simulink library "tp333079"  (Simulink 5.0)
values from neighbouring files (symbols this model uses):
  b = 1    [main_flock3.m]    (also in main_flock4.m; params_flocking_ros.m)
undefined symbols (not defined in the file or in its folder): AC, AlphaBnd, BetaBnd, CDda, CDde, CDdf, CDdr, CDM, CDmin, CGempty, CGgross, CL0, CLa, CLalphadot, Clbeta, Clda, CLde, CLdf, Cldr, CLM, CLmind, Clp, CLq, Clr, Cm0, Cma, Cmalphadot, Cmde, Cmdf, CmM, Cmq, Cnbeta, Cnda, Cndr, Cnp, Cnr, CP, CT, CYbeta, CYda, CYdr, CYp, CYr, Displacement, dmy, Engine, EulerIni, FuelFlow, FuelIni, J, Jempty, Jeng, Jgross, Jprop, MAC, MAP, MAPLim, MassIni, MaxPower, mempty ... (+26)
libraries: aerosimlib x325, simulink3 x42
(part 10 of 11)

== system tp333079/FlightGear-Compatible/Complete Aircraft/CESSNA-182/Aerodynamics/Yaw ==
  Control : Inport  Port=1  PortDimensions=[4 1]  SampleTime=-1  DataType=auto
      settings: SignalType=auto
  WindAxesVel : Inport  Port=2  PortDimensions=[3 1]  SampleTime=-1  DataType=auto
      settings: SignalType=auto
  AngularRates : Inport  Port=3  PortDimensions=[3 1]  SampleTime=-1  DataType=auto
      settings: SignalType=auto
  2 : Gain  Gain=2  Multiplication=Element-wise(K.*u)  SaturateOnIntegerOverflow=on
  Cn aileron : Subsystem  BlockChoice=Vector  SimViewingDevice=off
      link override Value: Value=AC.Aerodynamics.Yaw.Cnda
      link override Vector: Vector=AC.Aerodynamics.Yaw.CnDa
      settings: AttributesFormatString=%<BlockChoice>  TemplateBlock=aerosimlib/FlightGear-Compatible/Aerodynamics/Coefficient  MemberBlocks=Table,Value,Vector  Permissions=ReadWrite  RTWFcnNameOpts=Auto  RTWFileNameOpts=Auto
  Cn beta : Subsystem  BlockChoice=Vector  SimViewingDevice=off
      link override Value: Value=AC.Aerodynamics.Lift.Basic.kCLge
      link override Vector: Vector=AC.Aerodynamics.Yaw.Cnb
      settings: AttributesFormatString=%<BlockChoice>  TemplateBlock=aerosimlib/FlightGear-Compatible/Aerodynamics/Coefficient  MemberBlocks=Table,Value,Vector  Permissions=ReadWrite  RTWFcnNameOpts=Auto  RTWFileNameOpts=Auto
  Cn rudder : Subsystem  BlockChoice=Vector  SimViewingDevice=off
      link override Value: Value=AC.Aerodynamics.Yaw.Cndr
      link override Vector: Vector=AC.Aerodynamics.Yaw.CnDr
      settings: AttributesFormatString=%<BlockChoice>  TemplateBlock=aerosimlib/FlightGear-Compatible/Aerodynamics/Coefficient  MemberBlocks=Table,Value,Vector  Permissions=ReadWrite  RTWFcnNameOpts=Auto  RTWFileNameOpts=Auto
  Cn*b/(2V) : Product  Inputs=**/  Multiplication=Element-wise(.*)  SaturateOnIntegerOverflow=on
  Cnb*b{,1..4} (5 alike) : Product  Inputs=2  Multiplication=Element-wise(.*)  SaturateOnIntegerOverflow=on
  Cnp : Subsystem  BlockChoice=Vector  SimViewingDevice=off
      link override Value: Value=AC.Aerodynamics.Yaw.Cnp
      link override Vector: Vector=AC.Aerodynamics.Yaw.Cnp
      settings: AttributesFormatString=%<BlockChoice>  TemplateBlock=aerosimlib/FlightGear-Compatible/Aerodynamics/Coefficient  MemberBlocks=Table,Value,Vector  Permissions=ReadWrite  RTWFcnNameOpts=Auto  RTWFileNameOpts=Auto
  Cnr : Subsystem  BlockChoice=Vector  SimViewingDevice=off
      link override Value: Value=AC.Aerodynamics.Yaw.Cnr
      link override Vector: Vector=AC.Aerodynamics.Yaw.Cnr
      settings: AttributesFormatString=%<BlockChoice>  TemplateBlock=aerosimlib/FlightGear-Compatible/Aerodynamics/Coefficient  MemberBlocks=Table,Value,Vector  Permissions=ReadWrite  RTWFcnNameOpts=Auto  RTWFileNameOpts=Auto
  Demux : Demux  Outputs=4  BusSelectionMode=off
  Demux1 : Demux  Outputs=3  BusSelectionMode=off
  Demux3 : Demux  Outputs=3  BusSelectionMode=off
  Sum : Sum  Inputs=++  SaturateOnIntegerOverflow=on
  Sum1 : Sum  Inputs=++++  SaturateOnIntegerOverflow=on
  Terminator2 : Terminator
  Terminator3 : Terminator
  Terminator4 : Terminator
  Wing span : Constant  Value=AC.Metrics.WingSpan
  Cn : Outport  Port=1
  wires:
  Demux3/3 -> Cnb*b4/2
  Demux3/1 -> Cnb*b3/2
  Demux/4 -> Cnb*b2/2
  Demux/3 -> Cnb*b1/2
  Cnb*b2/1 -> Sum1/3
  Cnb*b1/1 -> Sum1/2
  Cnb*b3/1 -> Sum/1
  Cnb*b4/1 -> Sum/2
  Cnr/1(Coeff) -> Cnb*b4/1
  Cnp/1(Coeff) -> Cnb*b3/1
  Cn rudder/1(Coeff) -> Cnb*b2/1
  Cn aileron/1(Coeff) -> Cnb*b1/1
  Demux1/2 -> Cnb*b/2
  Cn beta/1(Coeff) -> Cnb*b/1
  Cnb*b/1 -> Sum1/1
  Cn*b/(2V)/1 -> Sum1/4
  Demux/2 -> Terminator3/1
  Demux/1 -> Terminator2/1
  Demux1/3 -> Cnp/1(RowParam), Cnr/1(RowParam), Cn rudder/1(RowParam), Cn aileron/1(RowParam), Cn beta/1(RowParam)
  Demux3/2 -> Terminator4/1
  Demux1/1 -> 2/1
  Sum/1 -> Cn*b/(2V)/1
  2/1 -> Cn*b/(2V)/3
  Wing span/1 -> Cn*b/(2V)/2
  WindAxesVel/1 -> Demux1/1
  Control/1 -> Demux/1
  AngularRates/1 -> Demux3/1
  Sum1/1 -> Cn/1

== system tp333079/FlightGear-Compatible/Complete Aircraft/CESSNA-310/Aerodynamics/Drag ==
  Control : Inport  Port=1  PortDimensions=[4 1]  SampleTime=-1  DataType=auto
      settings: SignalType=auto
  WindAxesVel : Inport  Port=2  PortDimensions=[3 1]  SampleTime=-1  DataType=auto
      settings: SignalType=auto
  Gear : Inport  Port=3  PortDimensions=1  SampleTime=-1  DataType=auto
      settings: SignalType=auto
  CD alpha : Subsystem  BlockChoice=Vector  SimViewingDevice=off
      link override Table: Table=AC.Aerodynamics.Drag.Basic.CDwbh
      link override Value: Value=AC.Aerodynamics.Lift.Basic.kCLge
      link override Vector: Vector=AC.Aerodynamics.Drag.CDalpha
      settings: AttributesFormatString=%<BlockChoice>  TemplateBlock=aerosimlib/FlightGear-Compatible/Aerodynamics/Coefficient  MemberBlocks=Table,Value,Vector  Permissions=ReadWrite  RTWFcnNameOpts=Auto  RTWFileNameOpts=Auto
  CD beta : Subsystem  BlockChoice=Value  SimViewingDevice=off
      link override Value: Value=AC.Aerodynamics.Drag.CDbeta
      settings: AttributesFormatString=%<BlockChoice>  TemplateBlock=aerosimlib/FlightGear-Compatible/Aerodynamics/Coefficient  MemberBlocks=Table,Value,Vector  Permissions=ReadWrite  RTWFcnNameOpts=Auto  RTWFileNameOpts=Auto
  CD elevator : Subsystem  BlockChoice=Value  SimViewingDevice=off
      link override Value: Value=AC.Aerodynamics.Drag.CDDe
      settings: AttributesFormatString=%<BlockChoice>  TemplateBlock=aerosimlib/FlightGear-Compatible/Aerodynamics/Coefficient  MemberBlocks=Table,Value,Vector  Permissions=ReadWrite  RTWFcnNameOpts=Auto  RTWFileNameOpts=Auto
  CD flap : Subsystem  BlockChoice=Vector  SimViewingDevice=off
      link override Table: Table=AC.Aerodynamics.Drag.CDDf
      link override Value: Value=AC.Aerodynamics.Lift.Basic.kCLge
      link override Vector: Vector=AC.Aerodynamics.Drag.CDDf
      settings: AttributesFormatString=%<BlockChoice>  TemplateBlock=aerosimlib/FlightGear-Compatible/Aerodynamics/Coefficient  MemberBlocks=Table,Value,Vector  Permissions=ReadWrite  RTWFcnNameOpts=Auto  RTWFileNameOpts=Auto
  CD gear : Subsystem  BlockChoice=Value  SimViewingDevice=off
      link override Value: Value=AC.Aerodynamics.Drag.CDgear
      settings: AttributesFormatString=%<BlockChoice>  TemplateBlock=aerosimlib/FlightGear-Compatible/Aerodynamics/Coefficient  MemberBlocks=Table,Value,Vector  Permissions=ReadWrite  RTWFcnNameOpts=Auto  RTWFileNameOpts=Auto
  CDo : Constant  Value=AC.Aerodynamics.Drag.CDo.Data
  Demux : Demux  Outputs=4  BusSelectionMode=off
  Demux1 : Demux  Outputs=3  BusSelectionMode=off
  Sum : Sum  Inputs=++  SaturateOnIntegerOverflow=on
  Sum1 : Sum  Inputs=+++++  SaturateOnIntegerOverflow=on
  Terminator : Terminator
  Terminator1 : Terminator
  Terminator5 : Terminator
  CD : Outport  Port=1
  wires:
  Gear/1 -> CD gear/1(RowParam)
  CD gear/1(Coeff) -> Sum1/5
  Demux/2 -> CD elevator/1(RowParam)
  WindAxesVel/1 -> Demux1/1
  Control/1 -> Demux/1
  Demux/3 -> Terminator/1
  Demux/4 -> Terminator1/1
  Demux1/3 -> CD alpha/1(RowParam)
  CD alpha/1(Coeff) -> Sum/1
  CD flap/1(Coeff) -> Sum/2
  Sum/1 -> Sum1/1
  CDo/1 -> Sum1/2
  CD elevator/1(Coeff) -> Sum1/3
  Sum1/1 -> CD/1
  Demux1/1 -> Terminator5/1
  Demux1/2 -> CD beta/1(RowParam)
  Demux/1 -> CD flap/1(RowParam)
  CD beta/1(Coeff) -> Sum1/4

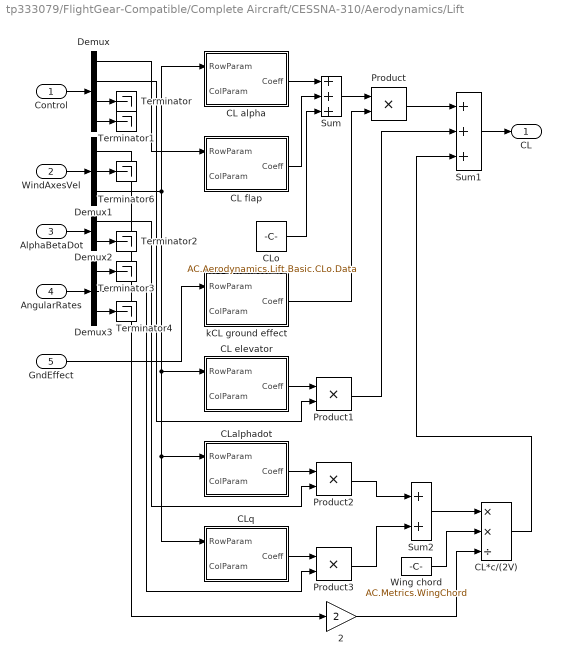
== system tp333079/FlightGear-Compatible/Complete Aircraft/CESSNA-310/Aerodynamics/Lift ==
  Control : Inport  Port=1  PortDimensions=[4 1]  SampleTime=-1  DataType=auto
      settings: SignalType=auto
  WindAxesVel : Inport  Port=2  PortDimensions=[3 1]  SampleTime=-1  DataType=auto
      settings: SignalType=auto
  AlphaBetaDot : Inport  Port=3  PortDimensions=[2 1]  SampleTime=-1  DataType=auto
      settings: SignalType=auto
  AngularRates : Inport  Port=4  PortDimensions=[3 1]  SampleTime=-1  DataType=auto
      settings: SignalType=auto
  GndEffect : Inport  Port=5  PortDimensions=1  SampleTime=-1  DataType=auto
      settings: SignalType=auto
  2 : Gain  Gain=2  Multiplication=Element-wise(K.*u)  SaturateOnIntegerOverflow=on
  CL alpha : Subsystem  BlockChoice=Vector  SimViewingDevice=off
      link override Table: Table=AC.Aerodynamics.Lift.Basic.CLalpha
      link override Value: Value=AC.Aerodynamics.Lift.Basic.kCLge
      link override Vector: Vector=AC.Aerodynamics.Lift.Basic.CLalpha
      settings: AttributesFormatString=%<BlockChoice>  TemplateBlock=aerosimlib/FlightGear-Compatible/Aerodynamics/Coefficient  MemberBlocks=Table,Value,Vector  Permissions=ReadWrite  RTWFcnNameOpts=Auto  RTWFileNameOpts=Auto
  CL elevator : Subsystem  BlockChoice=Vector  SimViewingDevice=off
      link override Value: Value=AC.Aerodynamics.Lift.CLDe
      link override Vector: Vector=AC.Aerodynamics.Lift.CLDe
      settings: AttributesFormatString=%<BlockChoice>  TemplateBlock=aerosimlib/FlightGear-Compatible/Aerodynamics/Coefficient  MemberBlocks=Table,Value,Vector  Permissions=ReadWrite  RTWFcnNameOpts=Auto  RTWFileNameOpts=Auto
  CL flap : Subsystem  BlockChoice=Vector  SimViewingDevice=off
      link override Value: Value=AC.Aerodynamics.Lift.Basic.kCLge
      link override Vector: Vector=AC.Aerodynamics.Lift.Basic.CLDf
      settings: AttributesFormatString=%<BlockChoice>  TemplateBlock=aerosimlib/FlightGear-Compatible/Aerodynamics/Coefficient  MemberBlocks=Table,Value,Vector  Permissions=ReadWrite  RTWFcnNameOpts=Auto  RTWFileNameOpts=Auto
  CL*c/(2V) : Product  Inputs=**/  Multiplication=Element-wise(.*)  SaturateOnIntegerOverflow=on
  CLalphadot : Subsystem  BlockChoice=Vector  SimViewingDevice=off
      link override Value: Value=AC.Aerodynamics.Lift.CLadot
      link override Vector: Vector=AC.Aerodynamics.Lift.CLadot
      settings: AttributesFormatString=%<BlockChoice>  TemplateBlock=aerosimlib/FlightGear-Compatible/Aerodynamics/Coefficient  MemberBlocks=Table,Value,Vector  Permissions=ReadWrite  RTWFcnNameOpts=Auto  RTWFileNameOpts=Auto
  CLo : Constant  Value=AC.Aerodynamics.Lift.Basic.CLo.Data
  CLq : Subsystem  BlockChoice=Vector  SimViewingDevice=off
      link override Value: Value=AC.Aerodynamics.Lift.CLq
      link override Vector: Vector=AC.Aerodynamics.Lift.CLq
      settings: AttributesFormatString=%<BlockChoice>  TemplateBlock=aerosimlib/FlightGear-Compatible/Aerodynamics/Coefficient  MemberBlocks=Table,Value,Vector  Permissions=ReadWrite  RTWFcnNameOpts=Auto  RTWFileNameOpts=Auto
  Demux : Demux  Outputs=4  BusSelectionMode=off
  Demux1 : Demux  Outputs=3  BusSelectionMode=off
  Demux2 : Demux  Outputs=2  BusSelectionMode=off
  Demux3 : Demux  Outputs=3  BusSelectionMode=off
  Product{,1..3} (4 alike) : Product  Inputs=2  Multiplication=Element-wise(.*)  SaturateOnIntegerOverflow=on
  Sum : Sum  Inputs=+++  SaturateOnIntegerOverflow=on
  Sum1 : Sum  Inputs=+++  SaturateOnIntegerOverflow=on
  Sum2 : Sum  Inputs=++  SaturateOnIntegerOverflow=on
  Terminator{,1..4,6} (6 alike) : Terminator
  Wing chord : Constant  Value=AC.Metrics.WingChord
  kCL ground effect : Subsystem  BlockChoice=Vector  SimViewingDevice=off
      link override Value: Value=AC.Aerodynamics.Lift.Basic.kCLge
      link override Vector: Vector=AC.Aerodynamics.Lift.Basic.kCLge
      settings: AttributesFormatString=%<BlockChoice>  TemplateBlock=aerosimlib/FlightGear-Compatible/Aerodynamics/Coefficient  MemberBlocks=Table,Value,Vector  Permissions=ReadWrite  RTWFcnNameOpts=Auto  RTWFileNameOpts=Auto
  CL : Outport  Port=1
  wires:
  Demux3/2 -> Product3/2
  Demux2/1 -> Product2/2
  Demux/2 -> Product1/2
  Product1/1 -> Sum1/2
  Product2/1 -> Sum2/1
  Product3/1 -> Sum2/2
  CLq/1(Coeff) -> Product3/1
  CLalphadot/1(Coeff) -> Product2/1
  CL elevator/1(Coeff) -> Product1/1
  CLo/1 -> Sum/3
  CL*c/(2V)/1 -> Sum1/3
  Sum2/1 -> CL*c/(2V)/1
  Wing chord/1 -> CL*c/(2V)/2
  2/1 -> CL*c/(2V)/3
  GndEffect/1 -> kCL ground effect/1(RowParam)
  Demux1/2 -> Terminator6/1
  Demux1/1 -> 2/1
  Sum1/1 -> CL/1
  Product/1 -> Sum1/1
  kCL ground effect/1(Coeff) -> Product/2
  Sum/1 -> Product/1
  CL flap/1(Coeff) -> Sum/2
  CL alpha/1(Coeff) -> Sum/1
  Demux3/3 -> Terminator4/1
  Demux3/1 -> Terminator3/1
  Demux2/2 -> Terminator2/1
  Demux1/3 -> CLq/1(RowParam), CLalphadot/1(RowParam), CL elevator/1(RowParam), CL alpha/1(RowParam)
  Demux/4 -> Terminator1/1
  Demux/3 -> Terminator/1
  Demux/1 -> CL flap/1(RowParam)
  AngularRates/1 -> Demux3/1
  AlphaBetaDot/1 -> Demux2/1
  Control/1 -> Demux/1
  WindAxesVel/1 -> Demux1/1

== system tp333079/FlightGear-Compatible/Complete Aircraft/CESSNA-310/Aerodynamics/Pitch ==
  Control : Inport  Port=1  PortDimensions=[4 1]  SampleTime=-1  DataType=auto
      settings: SignalType=auto
  WindAxesVel : Inport  Port=2  PortDimensions=[3 1]  SampleTime=-1  DataType=auto
      settings: SignalType=auto
  AlphaBetaDot : Inport  Port=3  PortDimensions=[2 1]  SampleTime=-1  DataType=auto
      settings: SignalType=auto
  AngularRates : Inport  Port=4  PortDimensions=[3 1]  SampleTime=-1  DataType=auto
      settings: SignalType=auto
  2 : Gain  Gain=2  Multiplication=Element-wise(K.*u)  SaturateOnIntegerOverflow=on
  Cm alpha : Subsystem  BlockChoice=Value  SimViewingDevice=off
      link override Table: Table=AC.Aerodynamics.Lift.Basic.CLwbh
      link override Value: Value=AC.Aerodynamics.Pitch.Cmalpha
      link override Vector: Vector=AC.Aerodynamics.Pitch.Cmalpha
      settings: AttributesFormatString=%<BlockChoice>  TemplateBlock=aerosimlib/FlightGear-Compatible/Aerodynamics/Coefficient  MemberBlocks=Table,Value,Vector  Permissions=ReadWrite  RTWFcnNameOpts=Auto  RTWFileNameOpts=Auto
  Cm elevator : Subsystem  BlockChoice=Value  SimViewingDevice=off
      link override Value: Value=AC.Aerodynamics.Pitch.CmDe
      link override Vector: Vector=AC.Aerodynamics.Pitch.CmDe
      settings: AttributesFormatString=%<BlockChoice>  TemplateBlock=aerosimlib/FlightGear-Compatible/Aerodynamics/Coefficient  MemberBlocks=Table,Value,Vector  Permissions=ReadWrite  RTWFcnNameOpts=Auto  RTWFileNameOpts=Auto
  Cm flap : Subsystem  BlockChoice=Vector  SimViewingDevice=off
      link override Value: Value=AC.Aerodynamics.Lift.Basic.kCLge
      link override Vector: Vector=AC.Aerodynamics.Pitch.CmDf
      settings: AttributesFormatString=%<BlockChoice>  TemplateBlock=aerosimlib/FlightGear-Compatible/Aerodynamics/Coefficient  MemberBlocks=Table,Value,Vector  Permissions=ReadWrite  RTWFcnNameOpts=Auto  RTWFileNameOpts=Auto
  Cm*c/(2V) : Product  Inputs=**/  Multiplication=Element-wise(.*)  SaturateOnIntegerOverflow=on
  Cmalphadot : Subsystem  BlockChoice=Value  SimViewingDevice=off
      link override Value: Value=AC.Aerodynamics.Pitch.Cmadot
      link override Vector: Vector=AC.Aerodynamics.Pitch.Cmadot
      settings: AttributesFormatString=%<BlockChoice>  TemplateBlock=aerosimlib/FlightGear-Compatible/Aerodynamics/Coefficient  MemberBlocks=Table,Value,Vector  Permissions=ReadWrite  RTWFcnNameOpts=Auto  RTWFileNameOpts=Auto
  Cmo : Constant  Value=AC.Aerodynamics.Pitch.Cmo.Data
  Cmq : Subsystem  BlockChoice=Value  SimViewingDevice=off
      link override Value: Value=AC.Aerodynamics.Pitch.Cmq
      link override Vector: Vector=AC.Aerodynamics.Pitch.Cmq
      settings: AttributesFormatString=%<BlockChoice>  TemplateBlock=aerosimlib/FlightGear-Compatible/Aerodynamics/Coefficient  MemberBlocks=Table,Value,Vector  Permissions=ReadWrite  RTWFcnNameOpts=Auto  RTWFileNameOpts=Auto
  Demux : Demux  Outputs=4  BusSelectionMode=off
  Demux1 : Demux  Outputs=3  BusSelectionMode=off
  Demux2 : Demux  Outputs=2  BusSelectionMode=off
  Demux3 : Demux  Outputs=3  BusSelectionMode=off
  Sum1 : Sum  Inputs=+++++  SaturateOnIntegerOverflow=on
  Sum2 : Sum  Inputs=++  SaturateOnIntegerOverflow=on
  Terminator{,1..4,6} (6 alike) : Terminator
  Wing chord : Constant  Value=AC.Metrics.WingChord
  Cm : Outport  Port=1
  wires:
  Cm elevator/1(Coeff) -> Sum1/4
  Cm alpha/1(Coeff) -> Sum1/1
  Cm*c/(2V)/1 -> Sum1/5
  Cmo/1 -> Sum1/3
  Cm flap/1(Coeff) -> Sum1/2
  Demux1/3 -> Cm alpha/1(RowParam)
  Demux1/1 -> 2/1
  Demux/1 -> Cm flap/1(RowParam)
  WindAxesVel/1 -> Demux1/1
  Control/1 -> Demux/1
  AlphaBetaDot/1 -> Demux2/1
  AngularRates/1 -> Demux3/1
  Demux/3 -> Terminator/1
  Demux/4 -> Terminator1/1
  Demux2/2 -> Terminator2/1
  Demux3/1 -> Terminator3/1
  Demux3/3 -> Terminator4/1
  Sum1/1 -> Cm/1
  Demux1/2 -> Terminator6/1
  2/1 -> Cm*c/(2V)/3
  Wing chord/1 -> Cm*c/(2V)/2
  Sum2/1 -> Cm*c/(2V)/1
  Demux/2 -> Cm elevator/1(RowParam)
  Cmalphadot/1(Coeff) -> Sum2/1
  Cmq/1(Coeff) -> Sum2/2
  Demux2/1 -> Cmalphadot/1(RowParam)
  Demux3/2 -> Cmq/1(RowParam)

== system tp333079/FlightGear-Compatible/Complete Aircraft/CESSNA-310/Aerodynamics/Roll ==
  Control : Inport  Port=1  PortDimensions=[4 1]  SampleTime=-1  DataType=auto
      settings: SignalType=auto
  WindAxesVel : Inport  Port=2  PortDimensions=[3 1]  SampleTime=-1  DataType=auto
      settings: SignalType=auto
  AngularRates : Inport  Port=3  PortDimensions=[3 1]  SampleTime=-1  DataType=auto
      settings: SignalType=auto
  2 : Gain  Gain=2  Multiplication=Element-wise(K.*u)  SaturateOnIntegerOverflow=on
  Cl aileron : Subsystem  BlockChoice=Value  SimViewingDevice=off
      link override Value: Value=AC.Aerodynamics.Roll.ClDa
      settings: AttributesFormatString=%<BlockChoice>  TemplateBlock=aerosimlib/FlightGear-Compatible/Aerodynamics/Coefficient  MemberBlocks=Table,Value,Vector  Permissions=ReadWrite  RTWFcnNameOpts=Auto  RTWFileNameOpts=Auto
  Cl beta : Subsystem  BlockChoice=Vector  SimViewingDevice=off
      link override Table: Table=AC.Aerodynamics.Roll.Clbeta
      link override Value: Value=AC.Aerodynamics.Lift.Basic.kCLge
      link override Vector: Vector=AC.Aerodynamics.Roll.Clbeta
      settings: AttributesFormatString=%<BlockChoice>  TemplateBlock=aerosimlib/FlightGear-Compatible/Aerodynamics/Coefficient  MemberBlocks=Table,Value,Vector  Permissions=ReadWrite  RTWFcnNameOpts=Auto  RTWFileNameOpts=Auto
  Cl rudder : Subsystem  BlockChoice=Value  SimViewingDevice=off
      link override Value: Value=AC.Aerodynamics.Roll.Cldr
      settings: AttributesFormatString=%<BlockChoice>  TemplateBlock=aerosimlib/FlightGear-Compatible/Aerodynamics/Coefficient  MemberBlocks=Table,Value,Vector  Permissions=ReadWrite  RTWFcnNameOpts=Auto  RTWFileNameOpts=Auto
  Cl*b/(2V) : Product  Inputs=**/  Multiplication=Element-wise(.*)  SaturateOnIntegerOverflow=on
  Clp : Subsystem  BlockChoice=Value  SimViewingDevice=off
      link override Value: Value=AC.Aerodynamics.Roll.Clp
      link override Vector: Vector=AC.Aerodynamics.Roll.Clp
      settings: AttributesFormatString=%<BlockChoice>  TemplateBlock=aerosimlib/FlightGear-Compatible/Aerodynamics/Coefficient  MemberBlocks=Table,Value,Vector  Permissions=ReadWrite  RTWFcnNameOpts=Auto  RTWFileNameOpts=Auto
  Clr : Subsystem  BlockChoice=Value  SimViewingDevice=off
      link override Value: Value=AC.Aerodynamics.Roll.Clr
      link override Vector: Vector=AC.Aerodynamics.Roll.Clr
      settings: AttributesFormatString=%<BlockChoice>  TemplateBlock=aerosimlib/FlightGear-Compatible/Aerodynamics/Coefficient  MemberBlocks=Table,Value,Vector  Permissions=ReadWrite  RTWFcnNameOpts=Auto  RTWFileNameOpts=Auto
  Demux : Demux  Outputs=4  BusSelectionMode=off
  Demux1 : Demux  Outputs=3  BusSelectionMode=off
  Demux3 : Demux  Outputs=3  BusSelectionMode=off
  Sum : Sum  Inputs=++  SaturateOnIntegerOverflow=on
  Sum1 : Sum  Inputs=++++  SaturateOnIntegerOverflow=on
  Terminator2 : Terminator
  Terminator3 : Terminator
  Terminator4 : Terminator
  Wing span : Constant  Value=AC.Metrics.WingSpan
  Cl : Outport  Port=1
  wires:
  Clr/1(Coeff) -> Sum/2
  Clp/1(Coeff) -> Sum/1
  Sum1/1 -> Cl/1
  AngularRates/1 -> Demux3/1
  Control/1 -> Demux/1
  WindAxesVel/1 -> Demux1/1
  Wing span/1 -> Cl*b/(2V)/2
  2/1 -> Cl*b/(2V)/3
  Sum/1 -> Cl*b/(2V)/1
  Demux1/1 -> 2/1
  Demux1/2 -> Cl beta/1(RowParam)
  Demux/3 -> Cl aileron/1(RowParam)
  Demux/4 -> Cl rudder/1(RowParam)
  Demux3/2 -> Terminator4/1
  Demux/1 -> Terminator2/1
  Demux/2 -> Terminator3/1
  Cl beta/1(Coeff) -> Sum1/1
  Cl aileron/1(Coeff) -> Sum1/2
  Cl rudder/1(Coeff) -> Sum1/3
  Cl*b/(2V)/1 -> Sum1/4
  Demux3/1 -> Clp/1(RowParam)
  Demux3/3 -> Clr/1(RowParam)

== system tp333079/FlightGear-Compatible/Complete Aircraft/CESSNA-310/Aerodynamics/Side ==
  Control : Inport  Port=1  PortDimensions=[4 1]  SampleTime=-1  DataType=auto
      settings: SignalType=auto
  WindAxesVel : Inport  Port=2  PortDimensions=[3 1]  SampleTime=-1  DataType=auto
      settings: SignalType=auto
  AngularRates : Inport  Port=3  PortDimensions=[3 1]  SampleTime=-1  DataType=auto
      settings: SignalType=auto
  2 : Gain  Gain=2  Multiplication=Element-wise(K.*u)  SaturateOnIntegerOverflow=on
  CY beta : Subsystem  BlockChoice=Vector  SimViewingDevice=off
      link override Value: Value=AC.Aerodynamics.Lift.Basic.kCLge
      link override Vector: Vector=AC.Aerodynamics.Side.CYbeta
      settings: AttributesFormatString=%<BlockChoice>  TemplateBlock=aerosimlib/FlightGear-Compatible/Aerodynamics/Coefficient  MemberBlocks=Table,Value,Vector  Permissions=ReadWrite  RTWFcnNameOpts=Auto  RTWFileNameOpts=Auto
  CY rudder : Subsystem  BlockChoice=Value  SimViewingDevice=off
      link override Value: Value=AC.Aerodynamics.Side.CYDr
      settings: AttributesFormatString=%<BlockChoice>  TemplateBlock=aerosimlib/FlightGear-Compatible/Aerodynamics/Coefficient  MemberBlocks=Table,Value,Vector  Permissions=ReadWrite  RTWFcnNameOpts=Auto  RTWFileNameOpts=Auto
  CY*b/(2V) : Product  Inputs=**/  Multiplication=Element-wise(.*)  SaturateOnIntegerOverflow=on
  CYp : Subsystem  BlockChoice=Value  SimViewingDevice=off
      link override Value: Value=AC.Aerodynamics.Side.CYp
      link override Vector: Vector=AC.Aerodynamics.Side.CYp
      settings: AttributesFormatString=%<BlockChoice>  TemplateBlock=aerosimlib/FlightGear-Compatible/Aerodynamics/Coefficient  MemberBlocks=Table,Value,Vector  Permissions=ReadWrite  RTWFcnNameOpts=Auto  RTWFileNameOpts=Auto
  CYr : Subsystem  BlockChoice=Value  SimViewingDevice=off
      link override Value: Value=AC.Aerodynamics.Side.CYr
      link override Vector: Vector=AC.Aerodynamics.Side.CYr
      settings: AttributesFormatString=%<BlockChoice>  TemplateBlock=aerosimlib/FlightGear-Compatible/Aerodynamics/Coefficient  MemberBlocks=Table,Value,Vector  Permissions=ReadWrite  RTWFcnNameOpts=Auto  RTWFileNameOpts=Auto
  Demux : Demux  Outputs=4  BusSelectionMode=off
  Demux1 : Demux  Outputs=3  BusSelectionMode=off
  Demux3 : Demux  Outputs=3  BusSelectionMode=off
  Sum : Sum  Inputs=++  SaturateOnIntegerOverflow=on
  Sum1 : Sum  Inputs=++++  SaturateOnIntegerOverflow=on
  Terminator2 : Terminator
  Terminator3 : Terminator
  Terminator4 : Terminator
  Wing span : Constant  Value=AC.Metrics.WingSpan
  CY : Outport  Port=1
  wires:
  Demux3/3 -> CYr/1(RowParam)
  CYr/1(Coeff) -> Sum/2
  CYp/1(Coeff) -> Sum/1
  CY*b/(2V)/1 -> Sum1/4
  CY rudder/1(Coeff) -> Sum1/3
  Demux/2 -> Terminator3/1
  Demux/1 -> Terminator2/1
  Demux3/2 -> Terminator4/1
  Demux/4 -> CY rudder/1(RowParam)
  Demux1/1 -> 2/1
  Sum/1 -> CY*b/(2V)/1
  2/1 -> CY*b/(2V)/3
  Wing span/1 -> CY*b/(2V)/2
  WindAxesVel/1 -> Demux1/1
  Control/1 -> Demux/1
  AngularRates/1 -> Demux3/1
  Sum1/1 -> CY/1
  CY beta/1(Coeff) -> Sum1/1
  Demux1/2 -> CY beta/1(RowParam)
  Demux3/1 -> CYp/1(RowParam)

== system tp333079/FlightGear-Compatible/Complete Aircraft/CESSNA-310/Aerodynamics/Yaw ==
  Control : Inport  Port=1  PortDimensions=[4 1]  SampleTime=-1  DataType=auto
      settings: SignalType=auto
  WindAxesVel : Inport  Port=2  PortDimensions=[3 1]  SampleTime=-1  DataType=auto
      settings: SignalType=auto
  AngularRates : Inport  Port=3  PortDimensions=[3 1]  SampleTime=-1  DataType=auto
      settings: SignalType=auto
  2 : Gain  Gain=2  Multiplication=Element-wise(K.*u)  SaturateOnIntegerOverflow=on
  Cn aileron : Subsystem  BlockChoice=Value  SimViewingDevice=off
      link override Value: Value=AC.Aerodynamics.Yaw.CnDa
      link override Vector: Vector=AC.Aerodynamics.Yaw.CnDa
      settings: AttributesFormatString=%<BlockChoice>  TemplateBlock=aerosimlib/FlightGear-Compatible/Aerodynamics/Coefficient  MemberBlocks=Table,Value,Vector  Permissions=ReadWrite  RTWFcnNameOpts=Auto  RTWFileNameOpts=Auto
  Cn beta : Subsystem  BlockChoice=Value  SimViewingDevice=off
      link override Value: Value=AC.Aerodynamics.Yaw.Cnbeta
      link override Vector: Vector=AC.Aerodynamics.Yaw.Cnb
      settings: AttributesFormatString=%<BlockChoice>  TemplateBlock=aerosimlib/FlightGear-Compatible/Aerodynamics/Coefficient  MemberBlocks=Table,Value,Vector  Permissions=ReadWrite  RTWFcnNameOpts=Auto  RTWFileNameOpts=Auto
  Cn rudder : Subsystem  BlockChoice=Value  SimViewingDevice=off
      link override Value: Value=AC.Aerodynamics.Yaw.CnDr
      link override Vector: Vector=AC.Aerodynamics.Yaw.CnDr
      settings: AttributesFormatString=%<BlockChoice>  TemplateBlock=aerosimlib/FlightGear-Compatible/Aerodynamics/Coefficient  MemberBlocks=Table,Value,Vector  Permissions=ReadWrite  RTWFcnNameOpts=Auto  RTWFileNameOpts=Auto
  Cn*b/(2V) : Product  Inputs=**/  Multiplication=Element-wise(.*)  SaturateOnIntegerOverflow=on
  Cnp : Subsystem  BlockChoice=Value  SimViewingDevice=off
      link override Value: Value=AC.Aerodynamics.Yaw.Cnp
      link override Vector: Vector=AC.Aerodynamics.Yaw.Cnp
      settings: AttributesFormatString=%<BlockChoice>  TemplateBlock=aerosimlib/FlightGear-Compatible/Aerodynamics/Coefficient  MemberBlocks=Table,Value,Vector  Permissions=ReadWrite  RTWFcnNameOpts=Auto  RTWFileNameOpts=Auto
  Cnr : Subsystem  BlockChoice=Value  SimViewingDevice=off
      link override Value: Value=AC.Aerodynamics.Yaw.Cnr
      link override Vector: Vector=AC.Aerodynamics.Yaw.Cnr
      settings: AttributesFormatString=%<BlockChoice>  TemplateBlock=aerosimlib/FlightGear-Compatible/Aerodynamics/Coefficient  MemberBlocks=Table,Value,Vector  Permissions=ReadWrite  RTWFcnNameOpts=Auto  RTWFileNameOpts=Auto
  Demux : Demux  Outputs=4  BusSelectionMode=off
  Demux1 : Demux  Outputs=3  BusSelectionMode=off
  Demux3 : Demux  Outputs=3  BusSelectionMode=off
  Sum : Sum  Inputs=++  SaturateOnIntegerOverflow=on
  Sum1 : Sum  Inputs=++++  SaturateOnIntegerOverflow=on
  Terminator2 : Terminator
  Terminator3 : Terminator
  Terminator4 : Terminator
  Wing span : Constant  Value=AC.Metrics.WingSpan
  Cn : Outport  Port=1
  wires:
  Demux/4 -> Cn rudder/1(RowParam)
  Cn aileron/1(Coeff) -> Sum1/2
  Cnr/1(Coeff) -> Sum/2
  Cnp/1(Coeff) -> Sum/1
  Cn rudder/1(Coeff) -> Sum1/3
  Cn*b/(2V)/1 -> Sum1/4
  Demux/2 -> Terminator3/1
  Demux/1 -> Terminator2/1
  Demux3/2 -> Terminator4/1
  Demux1/1 -> 2/1
  Sum/1 -> Cn*b/(2V)/1
  2/1 -> Cn*b/(2V)/3
  Wing span/1 -> Cn*b/(2V)/2
  WindAxesVel/1 -> Demux1/1
  Control/1 -> Demux/1
  AngularRates/1 -> Demux3/1
  Sum1/1 -> Cn/1
  Demux/3 -> Cn aileron/1(RowParam)
  Cn beta/1(Coeff) -> Sum1/1
  Demux1/2 -> Cn beta/1(RowParam)
  Demux3/1 -> Cnp/1(RowParam)
  Demux3/3 -> Cnr/1(RowParam)

== system tp333079/FlightGear-Compatible/Propulsion/Engine/Piston/AirFlow Model ==
  MAP : Inport  Port=1  PortDimensions=-1  SampleTime=-1  DataType=auto
      settings: SignalType=auto
  RPM : Inport  Port=2  PortDimensions=-1  SampleTime=-1  DataType=auto
      settings: SignalType=auto
  rho : Inport  Port=3  PortDimensions=-1  SampleTime=-1  DataType=auto
      settings: SignalType=auto
  p : Inport  Port=4  PortDimensions=-1  SampleTime=-1  DataType=auto
      settings: SignalType=auto
  1/2 : Gain  Gain=1/2  Multiplication=Element-wise(K.*u)  SaturateOnIntegerOverflow=on
  Displacement : Constant  Value=Disp/(100)^3
  Product : Product  Inputs=2  Multiplication=Element-wise(.*)  SaturateOnIntegerOverflow=on
  Product1 : Product  Inputs=3  Multiplication=Element-wise(.*)  SaturateOnIntegerOverflow=on
  Product2 : Product  Inputs=**/  Multiplication=Element-wise(.*)  SaturateOnIntegerOverflow=on
  Volumetric eff : Constant  Value=VolEff
  rot/sec : Gain  Gain=1/60  Multiplication=Element-wise(K.*u)  SaturateOnIntegerOverflow=on
  AirFlow : Outport  Port=1
  wires:
  Product1/1 -> AirFlow/1
  Product2/1 -> Product1/3
  p/1 -> Product2/3
  MAP/1 -> Product2/2
  rho/1 -> Product2/1
  Volumetric eff/1 -> Product1/2
  1/2/1 -> Product1/1
  Product/1 -> 1/2/1
  Displacement/1 -> Product/2
  rot/sec/1 -> Product/1
  RPM/1 -> rot/sec/1

== system tp333079/FlightGear-Compatible/Propulsion/Engine/Piston/FG Piston Engine ==
  Thr : Inport  Port=1  PortDimensions=1  SampleTime=-1  DataType=double
      settings: SignalType=auto
  Mix : Inport  Port=2  PortDimensions=1  SampleTime=-1  DataType=double
      settings: SignalType=auto
  Omega : Inport  Port=3  PortDimensions=1  SampleTime=-1  DataType=double
      settings: SignalType=auto
  p : Inport  Port=4  PortDimensions=1  SampleTime=-1  DataType=double
      settings: SignalType=auto
  T : Inport  Port=5  PortDimensions=1  SampleTime=-1  DataType=double
      settings: SignalType=auto
  rho : Inport  Port=6  PortDimensions=1  SampleTime=-1  DataType=double
      settings: SignalType=auto
  AirFlow Model : aerosimlib/FlightGear-Compatible/Propulsion/Engine/Piston/AirFlow Model  VolEff=0.8  Disp=Eng.Param.Displacement
  Engine torque : Product  Inputs=*/  Multiplication=Element-wise(.*)  SaturateOnIntegerOverflow=on
  Engine  BSFC : Product  Inputs=*/  Multiplication=Element-wise(.*)  SaturateOnIntegerOverflow=on
  FuelFlow Model : aerosimlib/FlightGear-Compatible/Propulsion/Engine/Piston/FuelFlow Model  pSL=pSL
  Intake Model : aerosimlib/FlightGear-Compatible/Propulsion/Engine/Piston/Intake Model  MAPLim=Eng.Param.MAPLim  pSL=pSL
  Power Model : aerosimlib/FlightGear-Compatible/Propulsion/Engine/Piston/Power Model  TSL=TSL  MaxPower=Eng.Param.MaxPower  Mixture=[14.7/1.6 10 11 12 13 14 15 16 17 18 19 20 14.7/0.6]  PowerMixCor=[78 86 93 98 100 99 96.4 92.5 88 83 78.5 74 58]
  rad/s 2 RPM : aerosimlib/Unit Conversion/Angular velocity/rad//s 2 RPM
  MAP : Outport  Port=1
  AirFlow : Outport  Port=2
  FuelFlow : Outport  Port=3
  BSFC : Outport  Port=4
  Power : Outport  Port=5
  Torque : Outport  Port=6
  wires:
  Power Model/1 -> Engine torque/1, Engine  BSFC/2, Power/1
  FuelFlow Model/2 -> FuelFlow/1, Engine  BSFC/1
  Mix/1 -> FuelFlow Model/1
  rho/1 -> AirFlow Model/3
  T/1 -> Power Model/3
  FuelFlow Model/1 -> Power Model/4
  AirFlow Model/1 -> AirFlow/1, FuelFlow Model/3
  rad/s 2 RPM/1 -> Power Model/2, AirFlow Model/2
  Intake Model/1 -> MAP/1, Power Model/1, AirFlow Model/1
  Omega/1 -> Engine torque/2, rad/s 2 RPM/1
  Engine  BSFC/1 -> BSFC/1
  Engine torque/1 -> Torque/1
  Thr/1 -> Intake Model/1
  p/1 -> AirFlow Model/4, FuelFlow Model/2, Intake Model/2

== system tp333079/FlightGear-Compatible/Propulsion/Engine/Piston/FuelFlow Model ==
  Mix : Inport  Port=1  PortDimensions=-1  SampleTime=-1  DataType=auto
      settings: SignalType=auto
  p : Inport  Port=2  PortDimensions=-1  SampleTime=-1  DataType=auto
      settings: SignalType=auto
  AirFlow : Inport  Port=3  PortDimensions=-1  SampleTime=-1  DataType=auto
      settings: SignalType=auto
  Gain : Gain  Gain=1.3  Multiplication=Element-wise(K.*u)  SaturateOnIntegerOverflow=on
  Product : Product  Inputs=**/  Multiplication=Element-wise(.*)  SaturateOnIntegerOverflow=on
  Product1 : Product  Inputs=**/  Multiplication=Element-wise(.*)  SaturateOnIntegerOverflow=on
  Sea-level pressure : Constant  Value=pSL
  coef : Constant  Value=14.7
  EquivRatio : Outport  Port=1
  FuelFlow : Outport  Port=2
  wires:
  Product1/1 -> FuelFlow/1
  coef/1 -> Product1/3
  AirFlow/1 -> Product1/2
  Product/1 -> Product1/1, EquivRatio/1
  p/1 -> Product/3
  Sea-level pressure/1 -> Product/2
  Gain/1 -> Product/1
  Mix/1 -> Gain/1

== system tp333079/FlightGear-Compatible/Propulsion/Engine/Piston/Intake Model ==
  Thr : Inport  Port=1  PortDimensions=1  SampleTime=-1  DataType=double
      settings: SignalType=auto
  p : Inport  Port=2  PortDimensions=1  SampleTime=-1  DataType=double
      settings: SignalType=auto
  Get MAP Altitude : Product  Inputs=**/  Multiplication=Element-wise(.*)  SaturateOnIntegerOverflow=on
  Get MAP Sea-level : Product  Inputs=2  Multiplication=Element-wise(.*)  SaturateOnIntegerOverflow=on
  MAP max : Constant  Value=MAPLim(2)
  MAP min : Constant  Value=MAPLim(1)
  Saturation : Saturate  UpperLimit=MAPLim(2)  LowerLimit=MAPLim(1)  LinearizeAsGain=on
  Sum : Sum  Inputs=|+-  SaturateOnIntegerOverflow=on
  Sum1 : Sum  Inputs=|++  SaturateOnIntegerOverflow=on
  p ambient : Constant  Value=pSL
  MAP : Outport  Port=1
  wires:
  Get MAP Altitude/1 -> MAP/1
  p ambient/1 -> Get MAP Altitude/3
  p/1 -> Get MAP Altitude/2
  Saturation/1 -> Get MAP Altitude/1
  MAP max/1 -> Sum/1
  Thr/1 -> Get MAP Sea-level/1
  MAP min/1 -> Sum/2, Sum1/2
  Sum/1 -> Get MAP Sea-level/2
  Get MAP Sea-level/1 -> Sum1/1
  Sum1/1 -> Saturation/1

== system tp333079/FlightGear-Compatible/Propulsion/Engine/Piston/Power Model ==
  MAP : Inport  Port=1  PortDimensions=-1  SampleTime=-1  DataType=auto
      settings: SignalType=auto
  RPM : Inport  Port=2  PortDimensions=-1  SampleTime=-1  DataType=auto
      settings: SignalType=auto
  T : Inport  Port=3  PortDimensions=-1  SampleTime=-1  DataType=auto
      settings: SignalType=auto
  EquivRatio : Inport  Port=4  PortDimensions=-1  SampleTime=-1  DataType=auto
      settings: SignalType=auto
  Gain : Gain  Gain=1/100  Multiplication=Element-wise(K.*u)  SaturateOnIntegerOverflow=on
  Gain1 : Gain  Gain=1/100  Multiplication=Element-wise(K.*u)  SaturateOnIntegerOverflow=on
  K2F : aerosimlib/Unit Conversion/Temperature/K2F
  K2F1 : aerosimlib/Unit Conversion/Temperature/K2F
  Look-Up Table : Lookup  InputValues=Mixture  OutputValues=PowerMixCor
  Math Function : Math  Operator=square  OutputSignalType=auto
  MaxPower : Constant  Value=MaxPower
  Pa2inHg : aerosimlib/Unit Conversion/Pressure/Pa2inHg
  Product{,1..3} (4 alike) : Product  Inputs=2  Multiplication=Element-wise(.*)  SaturateOnIntegerOverflow=on
  Product4 : Product  Inputs=3  Multiplication=Element-wise(.*)  SaturateOnIntegerOverflow=on
  Product5 : Product  Inputs=*/  Multiplication=Element-wise(.*)  SaturateOnIntegerOverflow=on
  Sum : Sum  Inputs=++-+  SaturateOnIntegerOverflow=on
  Sum1 : Sum  Inputs=|+-  SaturateOnIntegerOverflow=on
  T ambient : Constant  Value=TSL
  coef1 : Constant  Value=6e-9
  coef2 : Constant  Value=8e-4
  coef3 : Constant  Value=1
  coef4 : Constant  Value=7/120
  coef5 : Constant  Value=14.7
  Power : Outport  Port=1
  wires:
  coef5/1 -> Product5/1
  EquivRatio/1 -> Product5/2
  Product5/1 -> Look-Up Table/1
  Product4/1 -> Power/1
  MaxPower/1 -> Product4/3
  Gain/1 -> Product4/2
  Gain1/1 -> Product4/1
  Sum/1 -> Gain1/1
  Look-Up Table/1 -> Gain/1
  Product3/1 -> Sum/4
  coef4/1 -> Product3/2
  Sum1/1 -> Product3/1
  RPM/1 -> Product/2
  Pa2inHg/1 -> Product/1
  K2F/1 -> Sum1/2
  K2F1/1 -> Sum1/1
  T ambient/1 -> K2F1/1
  T/1 -> K2F/1
  coef3/1 -> Sum/3
  Product2/1 -> Sum/2
  Product1/1 -> Sum/1
  coef2/1 -> Product2/2
  coef1/1 -> Product1/2
  Math Function/1 -> Product1/1
  Product/1 -> Product2/1, Math Function/1
  MAP/1 -> Pa2inHg/1

== system tp333079/FlightGear-Compatible/Propulsion/Thruster/Propeller/FG Fixed-Pitch Propeller ==
  note: Sources
  note: Compute advance ratio
  note: Compute thrust force
  note: Interpolate propeller coefficients
  note: Compute torque
  Airspeed : Inport  Port=1  PortDimensions=1  SampleTime=-1  DataType=double
      settings: SignalType=auto
  rho : Inport  Port=2  PortDimensions=1  SampleTime=-1  DataType=double
      settings: SignalType=auto
  Omega : Inport  Port=3  PortDimensions=1  SampleTime=-1  DataType=double
      settings: SignalType=auto
  1/pi^2 : Math  Operator=pow  OutputSignalType=auto
  1/pi^3 : Math  Operator=pow  OutputSignalType=auto
  Advance Ratio : Product  Inputs=**//  Multiplication=Element-wise(.*)  SaturateOnIntegerOverflow=on
  Coeff of Power : Lookup  InputValues=Thr.Param.CoefPower(:,1)  OutputValues=Thr.Param.CoefPower(:,2)
  Coeff of Thrust : Lookup  InputValues=Thr.Param.CoefThrust(:,1)  OutputValues=Thr.Param.CoefThrust(:,2)
  Gain : Gain  Gain=4  Multiplication=Element-wise(K.*u)  SaturateOnIntegerOverflow=on
  Gain1 : Gain  Gain=-4  Multiplication=Element-wise(K.*u)  SaturateOnIntegerOverflow=on
  Mux : Mux  Inputs=3
  Omega^2 : Math  Operator=square  OutputSignalType=auto
  Pi : Constant  Value=pi
  Prop Radius : Constant  Value=Thr.Param.Diameter/2
  R^4 : Math  Operator=pow  OutputSignalType=auto
  R^5 : Math  Operator=pow  OutputSignalType=auto
  Thrust : Product  Inputs=5  Multiplication=Element-wise(.*)  SaturateOnIntegerOverflow=on
  Torque : Product  Inputs=5  Multiplication=Element-wise(.*)  SaturateOnIntegerOverflow=on
  exp : Constant  Value=-3
  exp1 : Constant  Value=4
  exp2 : Constant  Value=5
  exp3 : Constant  Value=-2
  Fprop : Outport  Port=1
  Mprop : Outport  Port=2
  PropCoeff : Outport  Port=3
  wires:
  exp3/1 -> 1/pi^2/2
  Coeff of Power/1 -> Mux/3, Torque/5
  Airspeed/1 -> Advance Ratio/2
  rho/1 -> Torque/2, Thrust/2
  Omega/1 -> Advance Ratio/3, Omega^2/1
  Pi/1 -> Advance Ratio/1, 1/pi^2/1, 1/pi^3/1
  Prop Radius/1 -> Advance Ratio/4, R^4/1, R^5/1
  Advance Ratio/1 -> Mux/1, Coeff of Power/1, Coeff of Thrust/1
  Omega^2/1 -> Torque/4, Thrust/4
  exp/1 -> 1/pi^3/2
  1/pi^2/1 -> Gain/1
  1/pi^3/1 -> Gain1/1
  exp1/1 -> R^4/2
  R^4/1 -> Thrust/3
  exp2/1 -> R^5/2
  R^5/1 -> Torque/3
  Gain/1 -> Thrust/1
  Gain1/1 -> Torque/1
  Coeff of Thrust/1 -> Mux/2, Thrust/5
  Thrust/1 -> Fprop/1
  Torque/1 -> Mprop/1
  Mux/1 -> PropCoeff/1

== system tp333079/FlightGear-Compatible/Propulsion/Thruster/Propeller/FG Variable-Pitch Propeller ==
  note: Sources
  note: Compute advance ratio
  note: Compute thrust force
  note: Interpolate propeller coefficients
  note: Compute torque
  Airspeed : Inport  Port=1  PortDimensions=1  SampleTime=-1  DataType=double
      settings: SignalType=auto
  rho : Inport  Port=2  PortDimensions=1  SampleTime=-1  DataType=double
      settings: SignalType=auto
  Omega : Inport  Port=3  PortDimensions=1  SampleTime=-1  DataType=double
      settings: SignalType=auto
  Pitch : Inport  Port=4  PortDimensions=1  SampleTime=-1  DataType=double
      settings: SignalType=auto
  1/pi^2 : Math  Operator=pow  OutputSignalType=auto
  1/pi^3 : Math  Operator=pow  OutputSignalType=auto
  Advance Ratio : Product  Inputs=**//  Multiplication=Element-wise(.*)  SaturateOnIntegerOverflow=on
  Coeff of Power : Lookup2D  RowIndex=Thr.Param.CoefPower(2:end,1)  ColumnIndex=Thr.Param.CoefPower(1,2:end)  OutputValues=Thr.Param.CoefPower(2:end,2:end)
  Coeff of Thrust : Lookup2D  RowIndex=Thr.Param.CoefThrust(2:end,1)  ColumnIndex=Thr.Param.CoefThrust(1,2:end)  OutputValues=Thr.Param.CoefThrust(2:end,2:end)
  Gain : Gain  Gain=4  Multiplication=Element-wise(K.*u)  SaturateOnIntegerOverflow=on
  Gain1 : Gain  Gain=-4  Multiplication=Element-wise(K.*u)  SaturateOnIntegerOverflow=on
  Mux : Mux  Inputs=3
  Omega^2 : Math  Operator=square  OutputSignalType=auto
  Pi : Constant  Value=pi
  Prop Radius : Constant  Value=Thr.Param.Diameter/2
  R^4 : Math  Operator=pow  OutputSignalType=auto
  R^5 : Math  Operator=pow  OutputSignalType=auto
  Thrust : Product  Inputs=5  Multiplication=Element-wise(.*)  SaturateOnIntegerOverflow=on
  Torque : Product  Inputs=5  Multiplication=Element-wise(.*)  SaturateOnIntegerOverflow=on
  exp : Constant  Value=-3
  exp1 : Constant  Value=4
  exp2 : Constant  Value=5
  exp3 : Constant  Value=-2
  Fprop : Outport  Port=1
  Mprop : Outport  Port=2
  PropCoeff : Outport  Port=3
  wires:
  Pitch/1 -> Coeff of Power/2, Coeff of Thrust/2
  exp3/1 -> 1/pi^2/2
  Coeff of Power/1 -> Mux/3, Torque/5
  Airspeed/1 -> Advance Ratio/2
  rho/1 -> Torque/2, Thrust/2
  Omega/1 -> Advance Ratio/3, Omega^2/1
  Pi/1 -> Advance Ratio/1, 1/pi^2/1, 1/pi^3/1
  Prop Radius/1 -> Advance Ratio/4, R^4/1, R^5/1
  Advance Ratio/1 -> Coeff of Power/1, Mux/1, Coeff of Thrust/1
  Omega^2/1 -> Torque/4, Thrust/4
  exp/1 -> 1/pi^3/2
  1/pi^2/1 -> Gain/1
  1/pi^3/1 -> Gain1/1
  exp1/1 -> R^4/2
  R^4/1 -> Thrust/3
  exp2/1 -> R^5/2
  R^5/1 -> Torque/3
  Gain/1 -> Thrust/1
  Gain1/1 -> Torque/1
  Coeff of Thrust/1 -> Mux/2, Thrust/5
  Thrust/1 -> Fprop/1
  Torque/1 -> Mprop/1
  Mux/1 -> PropCoeff/1

== system tp333079/FlightGear-Compatible/Complete Aircraft/CESSNA-172/Aerodynamics/Drag/CD alpha ==
  RowParam : Inport  Port=1  PortDimensions=-1  SampleTime=-1  DataType=auto
      settings: SignalType=auto
  ColParam : Inport  Port=2  PortDimensions=-1  SampleTime=-1  DataType=auto
      settings: SignalType=auto
  Table : aerosimlib/FlightGear-Compatible/Aerodynamics/Table  Table=AC.Aerodynamics.Drag.Basic.CDwbh
  Coeff : Outport  Port=1
  wires:
  Table/1 -> Coeff/1
  ColParam/1 -> Table/2
  RowParam/1 -> Table/1

== system tp333079/FlightGear-Compatible/Complete Aircraft/CESSNA-172/Aerodynamics/Drag/CD beta ==
  RowParam : Inport  Port=1  PortDimensions=-1  SampleTime=-1  DataType=auto
      settings: SignalType=auto
  ColParam : Inport  Port=2  PortDimensions=-1  SampleTime=-1  DataType=auto
      settings: SignalType=auto
  Value : aerosimlib/FlightGear-Compatible/Aerodynamics/Value  Value=AC.Aerodynamics.Drag.CDbeta
  term2 : Terminator
  Coeff : Outport  Port=1
  wires:
  ColParam/1 -> term2/1
  Value/1 -> Coeff/1
  RowParam/1 -> Value/1

== system tp333079/FlightGear-Compatible/Complete Aircraft/CESSNA-172/Aerodynamics/Drag/CD elevator ==
  RowParam : Inport  Port=1  PortDimensions=-1  SampleTime=-1  DataType=auto
      settings: SignalType=auto
  ColParam : Inport  Port=2  PortDimensions=-1  SampleTime=-1  DataType=auto
      settings: SignalType=auto
  Value : aerosimlib/FlightGear-Compatible/Aerodynamics/Value  Value=AC.Aerodynamics.Drag.CDDe
  term2 : Terminator
  Coeff : Outport  Port=1
  wires:
  ColParam/1 -> term2/1
  Value/1 -> Coeff/1
  RowParam/1 -> Value/1

== system tp333079/FlightGear-Compatible/Complete Aircraft/CESSNA-172/Aerodynamics/Drag/CD flap ==
  RowParam : Inport  Port=1  PortDimensions=-1  SampleTime=-1  DataType=auto
      settings: SignalType=auto
  ColParam : Inport  Port=2  PortDimensions=-1  SampleTime=-1  DataType=auto
      settings: SignalType=auto
  Vector : aerosimlib/FlightGear-Compatible/Aerodynamics/Vector  Vector=AC.Aerodynamics.Drag.Basic.CDDf
  term2 : Terminator
  Coeff : Outport  Port=1
  wires:
  ColParam/1 -> term2/1
  Vector/1 -> Coeff/1
  RowParam/1 -> Vector/1

== system tp333079/FlightGear-Compatible/Complete Aircraft/CESSNA-172/Aerodynamics/Drag/kCD ground effect ==
  RowParam : Inport  Port=1  PortDimensions=-1  SampleTime=-1  DataType=auto
      settings: SignalType=auto
  ColParam : Inport  Port=2  PortDimensions=-1  SampleTime=-1  DataType=auto
      settings: SignalType=auto
  Vector : aerosimlib/FlightGear-Compatible/Aerodynamics/Vector  Vector=AC.Aerodynamics.Drag.Basic.kCDge
  term2 : Terminator
  Coeff : Outport  Port=1
  wires:
  ColParam/1 -> term2/1
  Vector/1 -> Coeff/1
  RowParam/1 -> Vector/1

== system tp333079/FlightGear-Compatible/Complete Aircraft/CESSNA-172/Aerodynamics/Lift/CL alpha ==
  RowParam : Inport  Port=1  PortDimensions=-1  SampleTime=-1  DataType=auto
      settings: SignalType=auto
  ColParam : Inport  Port=2  PortDimensions=-1  SampleTime=-1  DataType=auto
      settings: SignalType=auto
  Table : aerosimlib/FlightGear-Compatible/Aerodynamics/Table  Table=AC.Aerodynamics.Lift.Basic.CLwbh
  Coeff : Outport  Port=1
  wires:
  RowParam/1 -> Table/1
  ColParam/1 -> Table/2
  Table/1 -> Coeff/1

== system tp333079/FlightGear-Compatible/Complete Aircraft/CESSNA-172/Aerodynamics/Lift/CL elevator ==
  RowParam : Inport  Port=1  PortDimensions=-1  SampleTime=-1  DataType=auto
      settings: SignalType=auto
  ColParam : Inport  Port=2  PortDimensions=-1  SampleTime=-1  DataType=auto
      settings: SignalType=auto
  Value : aerosimlib/FlightGear-Compatible/Aerodynamics/Value  Value=AC.Aerodynamics.Lift.CLDe
  term2 : Terminator
  Coeff : Outport  Port=1
  wires:
  RowParam/1 -> Value/1
  Value/1 -> Coeff/1
  ColParam/1 -> term2/1

== system tp333079/FlightGear-Compatible/Complete Aircraft/CESSNA-172/Aerodynamics/Lift/CL flap ==
  RowParam : Inport  Port=1  PortDimensions=-1  SampleTime=-1  DataType=auto
      settings: SignalType=auto
  ColParam : Inport  Port=2  PortDimensions=-1  SampleTime=-1  DataType=auto
      settings: SignalType=auto
  Vector : aerosimlib/FlightGear-Compatible/Aerodynamics/Vector  Vector=AC.Aerodynamics.Lift.Basic.CLDf
  term2 : Terminator
  Coeff : Outport  Port=1
  wires:
  RowParam/1 -> Vector/1
  Vector/1 -> Coeff/1
  ColParam/1 -> term2/1

== system tp333079/FlightGear-Compatible/Complete Aircraft/CESSNA-172/Aerodynamics/Lift/CLalphadot ==
  RowParam : Inport  Port=1  PortDimensions=-1  SampleTime=-1  DataType=auto
      settings: SignalType=auto
  ColParam : Inport  Port=2  PortDimensions=-1  SampleTime=-1  DataType=auto
      settings: SignalType=auto
  Value : aerosimlib/FlightGear-Compatible/Aerodynamics/Value  Value=AC.Aerodynamics.Lift.CLadot
  term2 : Terminator
  Coeff : Outport  Port=1
  wires:
  RowParam/1 -> Value/1
  Value/1 -> Coeff/1
  ColParam/1 -> term2/1

== system tp333079/FlightGear-Compatible/Complete Aircraft/CESSNA-172/Aerodynamics/Lift/CLq ==
  RowParam : Inport  Port=1  PortDimensions=-1  SampleTime=-1  DataType=auto
      settings: SignalType=auto
  ColParam : Inport  Port=2  PortDimensions=-1  SampleTime=-1  DataType=auto
      settings: SignalType=auto
  Value : aerosimlib/FlightGear-Compatible/Aerodynamics/Value  Value=AC.Aerodynamics.Lift.CLq
  term2 : Terminator
  Coeff : Outport  Port=1
  wires:
  RowParam/1 -> Value/1
  Value/1 -> Coeff/1
  ColParam/1 -> term2/1

== system tp333079/FlightGear-Compatible/Complete Aircraft/CESSNA-172/Aerodynamics/Lift/kCL ground effect ==
  RowParam : Inport  Port=1  PortDimensions=-1  SampleTime=-1  DataType=auto
      settings: SignalType=auto
  ColParam : Inport  Port=2  PortDimensions=-1  SampleTime=-1  DataType=auto
      settings: SignalType=auto
  Vector : aerosimlib/FlightGear-Compatible/Aerodynamics/Vector  Vector=AC.Aerodynamics.Lift.Basic.kCLge
  term2 : Terminator
  Coeff : Outport  Port=1
  wires:
  RowParam/1 -> Vector/1
  Vector/1 -> Coeff/1
  ColParam/1 -> term2/1

== system tp333079/FlightGear-Compatible/Complete Aircraft/CESSNA-172/Aerodynamics/Pitch/Cm alpha ==
  RowParam : Inport  Port=1  PortDimensions=-1  SampleTime=-1  DataType=auto
      settings: SignalType=auto
  ColParam : Inport  Port=2  PortDimensions=-1  SampleTime=-1  DataType=auto
      settings: SignalType=auto
  Value : aerosimlib/FlightGear-Compatible/Aerodynamics/Value  Value=AC.Aerodynamics.Pitch.Cmalpha
  term2 : Terminator
  Coeff : Outport  Port=1
  wires:
  RowParam/1 -> Value/1
  Value/1 -> Coeff/1
  ColParam/1 -> term2/1

== system tp333079/FlightGear-Compatible/Complete Aircraft/CESSNA-172/Aerodynamics/Pitch/Cm elevator ==
  RowParam : Inport  Port=1  PortDimensions=-1  SampleTime=-1  DataType=auto
      settings: SignalType=auto
  ColParam : Inport  Port=2  PortDimensions=-1  SampleTime=-1  DataType=auto
      settings: SignalType=auto
  Value : aerosimlib/FlightGear-Compatible/Aerodynamics/Value  Value=AC.Aerodynamics.Pitch.Cmde
  term2 : Terminator
  Coeff : Outport  Port=1
  wires:
  RowParam/1 -> Value/1
  Value/1 -> Coeff/1
  ColParam/1 -> term2/1

== system tp333079/FlightGear-Compatible/Complete Aircraft/CESSNA-172/Aerodynamics/Pitch/Cm flap ==
  RowParam : Inport  Port=1  PortDimensions=-1  SampleTime=-1  DataType=auto
      settings: SignalType=auto
  ColParam : Inport  Port=2  PortDimensions=-1  SampleTime=-1  DataType=auto
      settings: SignalType=auto
  Vector : aerosimlib/FlightGear-Compatible/Aerodynamics/Vector  Vector=AC.Aerodynamics.Pitch.Cmdf
  term2 : Terminator
  Coeff : Outport  Port=1
  wires:
  RowParam/1 -> Vector/1
  Vector/1 -> Coeff/1
  ColParam/1 -> term2/1

== system tp333079/FlightGear-Compatible/Complete Aircraft/CESSNA-172/Aerodynamics/Pitch/Cmalphadot ==
  RowParam : Inport  Port=1  PortDimensions=-1  SampleTime=-1  DataType=auto
      settings: SignalType=auto
  ColParam : Inport  Port=2  PortDimensions=-1  SampleTime=-1  DataType=auto
      settings: SignalType=auto
  Value : aerosimlib/FlightGear-Compatible/Aerodynamics/Value  Value=AC.Aerodynamics.Pitch.Cmadot
  term2 : Terminator
  Coeff : Outport  Port=1
  wires:
  RowParam/1 -> Value/1
  Value/1 -> Coeff/1
  ColParam/1 -> term2/1

== system tp333079/FlightGear-Compatible/Complete Aircraft/CESSNA-172/Aerodynamics/Pitch/Cmq ==
  RowParam : Inport  Port=1  PortDimensions=-1  SampleTime=-1  DataType=auto
      settings: SignalType=auto
  ColParam : Inport  Port=2  PortDimensions=-1  SampleTime=-1  DataType=auto
      settings: SignalType=auto
  Value : aerosimlib/FlightGear-Compatible/Aerodynamics/Value  Value=AC.Aerodynamics.Pitch.Cmq
  term2 : Terminator
  Coeff : Outport  Port=1
  wires:
  RowParam/1 -> Value/1
  Value/1 -> Coeff/1
  ColParam/1 -> term2/1
